simulink model "biquad_filter"  (R2022a)
settings: Solver=FixedStepDiscrete  StartTime=0.0  StopTime=10.0  RelTol=1e-3
PreLoadFcn:
  | addpath('C:\Users\Besic\Documents\MATLAB\hdlimport\biquad_filter');
CloseFcn:
  | addpath('C:\Users\Besic\Documents\MATLAB\hdlimport\biquad_filter');
  | rmpath('C:\Users\Besic\Documents\MATLAB\hdlimport\biquad_filter');
settings Model: DataTypeOverride=Off  Creator=Besic  LastModifiedBy=Besic
settings OptimizationCC: BlockReduction=off  ConditionallyExecuteInputs=off  DefaultParameterBehavior=Inlined  InheritOutputTypeSmallerThanSingle=on
settings DebuggingCC: AlgebraicLoopMsg=error  InheritedTsInSrcMsg=none  SingleTaskRateTransMsg=error
settings HardwareCC: ProdBitPerPointer=32  ProdBitPerSizeT=32  ProdBitPerPtrDiffT=32  ProdLargestAtomicFloat=None  ProdIntDivRoundTo=Undefined  ProdEndianess=Unspecified  ProdWordSize=32  ProdHWDeviceType=ASIC/FPGA->ASIC/FPGA  TargetBitPerPointer=64  TargetBitPerSizeT=64  TargetBitPerPtrDiffT=64  TargetLongLongMode=on  TargetIntDivRoundTo=Zero  TargetEndianess=LittleEndian  TargetWordSize=64  TargetHWDeviceType=Custom Processor->MATLAB Host Computer  ProdEqTarget=off

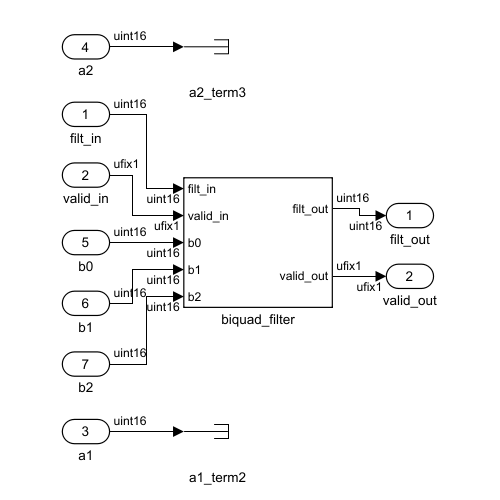
[thumbnail: Simulink's stored preview of the top-level diagram]
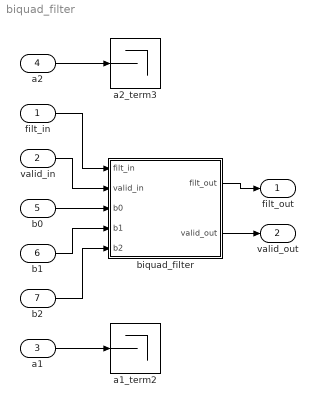
== system biquad_filter ==
  filt_in : Inport  OutDataTypeStr=uint16  SampleTime=-1
  valid_in : Inport  Port=2  OutDataTypeStr=fixdt(0, 1, 0)  SampleTime=-1
  a1 : Inport  Port=3  OutDataTypeStr=uint16  SampleTime=-1
  a2 : Inport  Port=4  OutDataTypeStr=uint16  SampleTime=-1
  b0 : Inport  Port=5  OutDataTypeStr=uint16  SampleTime=-1
  b1 : Inport  Port=6  OutDataTypeStr=uint16  SampleTime=-1
  b2 : Inport  Port=7  OutDataTypeStr=uint16  SampleTime=-1
  a1_term2 : Terminator
  a2_term3 : Terminator
  biquad_filter : Subsystem
  filt_out : Outport  OutDataTypeStr=uint16  SampleTime=-1
  valid_out : Outport  Port=2  OutDataTypeStr=fixdt(0, 1, 0)  SampleTime=-1
  wires:
  a1/1 -> a1_term2/1
  valid_in/1 -> biquad_filter/2(valid_in)
  biquad_filter/2(valid_out) -> valid_out/1
  biquad_filter/1(filt_out) -> filt_out/1
  b2/1 -> biquad_filter/5(b2)
  b1/1 -> biquad_filter/4(b1)
  b0/1 -> biquad_filter/3(b0)
  a2/1 -> a2_term3/1
  filt_in/1 -> biquad_filter/1(filt_in)

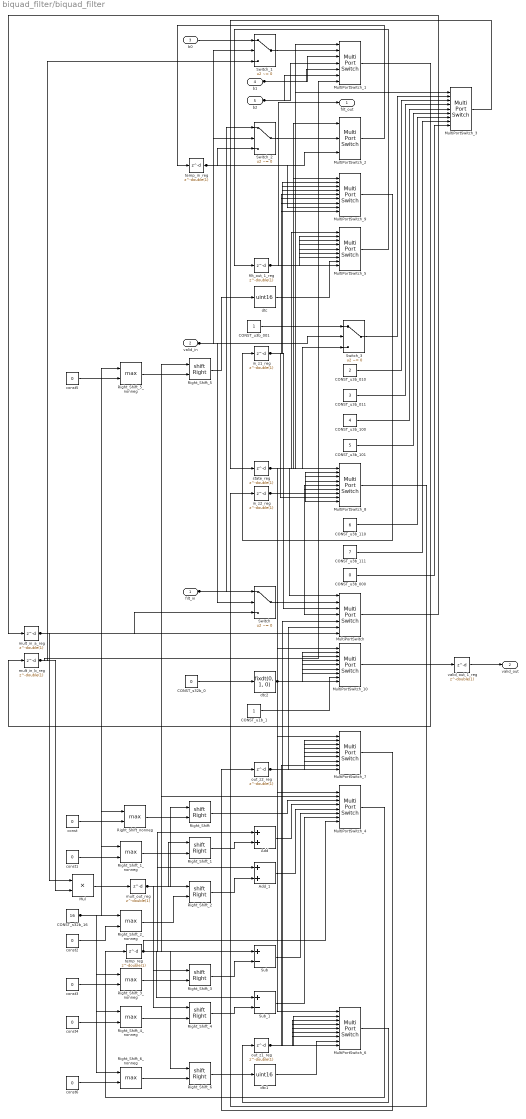
== system biquad_filter/biquad_filter ==
  filt_in : Inport  OutDataTypeStr=uint16  SampleTime=-1
  valid_in : Inport  Port=2  OutDataTypeStr=fixdt(0, 1, 0)  SampleTime=-1
  b0 : Inport  Port=3  OutDataTypeStr=uint16  SampleTime=-1
  b1 : Inport  Port=4  OutDataTypeStr=uint16  SampleTime=-1
  b2 : Inport  Port=5  OutDataTypeStr=uint16  SampleTime=-1
  Add : Sum  AccumDataTypeStr=uint32  OutDataTypeStr=uint32  SampleTime=-1
  Add_1 : Sum  AccumDataTypeStr=uint32  OutDataTypeStr=uint32  SampleTime=-1
  CONST_s32b_0 : Constant  Value=0  OutDataTypeStr=int32  SampleTime=-1
  CONST_s32b_16 : Constant  Value=16  OutDataTypeStr=int32  SampleTime=-1
  CONST_u1b_1 : Constant  OutDataTypeStr=fixdt(0, 1, 0)  SampleTime=-1
  CONST_u3b_000 : Constant  Value=0  OutDataTypeStr=fixdt(0, 3, 0)  SampleTime=-1
  CONST_u3b_001 : Constant  OutDataTypeStr=fixdt(0, 3, 0)  SampleTime=-1
  CONST_u3b_010 : Constant  Value=2  OutDataTypeStr=fixdt(0, 3, 0)  SampleTime=-1
  CONST_u3b_011 : Constant  Value=3  OutDataTypeStr=fixdt(0, 3, 0)  SampleTime=-1
  CONST_u3b_100 : Constant  Value=4  OutDataTypeStr=fixdt(0, 3, 0)  SampleTime=-1
  CONST_u3b_101 : Constant  Value=5  OutDataTypeStr=fixdt(0, 3, 0)  SampleTime=-1
  CONST_u3b_110 : Constant  Value=6  OutDataTypeStr=fixdt(0, 3, 0)  SampleTime=-1
  CONST_u3b_111 : Constant  Value=7  OutDataTypeStr=fixdt(0, 3, 0)  SampleTime=-1
  Mul : Product  Inputs=**  OutDataTypeStr=uint32  SampleTime=-1
  MultiPortSwitch : MultiPortSwitch  DataPortOrder=Zero-based contiguous  Inputs=6  DiagnosticForDefault=None  zeroidx=on  OutDataTypeStr=uint16  SampleTime=-1  SaturateOnIntegerOverflow=off  InputSameDT=off
  MultiPortSwitch_1 : MultiPortSwitch  DataPortOrder=Zero-based contiguous  Inputs=6  DiagnosticForDefault=None  zeroidx=on  OutDataTypeStr=uint16  SampleTime=-1  SaturateOnIntegerOverflow=off  InputSameDT=off
  MultiPortSwitch_10 : MultiPortSwitch  DataPortOrder=Zero-based contiguous  Inputs=8  DiagnosticForDefault=None  zeroidx=on  OutDataTypeStr=fixdt(0, 1, 0)  SampleTime=-1  SaturateOnIntegerOverflow=off  InputSameDT=off
  MultiPortSwitch_2 : MultiPortSwitch  DataPortOrder=Zero-based contiguous  Inputs=2  DiagnosticForDefault=None  zeroidx=on  OutDataTypeStr=uint16  SampleTime=-1  SaturateOnIntegerOverflow=off  InputSameDT=off
  MultiPortSwitch_3 : MultiPortSwitch  DataPortOrder=Zero-based contiguous  Inputs=8  DiagnosticForDefault=None  zeroidx=on  OutDataTypeStr=fixdt(0, 3, 0)  SampleTime=-1  SaturateOnIntegerOverflow=off  InputSameDT=off
  MultiPortSwitch_4 : MultiPortSwitch  DataPortOrder=Zero-based contiguous  Inputs=7  DiagnosticForDefault=None  zeroidx=on  OutDataTypeStr=uint32  SampleTime=-1  SaturateOnIntegerOverflow=off  InputSameDT=off
  MultiPortSwitch_{5..9} (5 alike) : MultiPortSwitch  DataPortOrder=Zero-based contiguous  Inputs=8  DiagnosticForDefault=None  zeroidx=on  OutDataTypeStr=uint16  SampleTime=-1  SaturateOnIntegerOverflow=off  InputSameDT=off
  Right_Shift : ArithShift  BitShiftNumberSource=Input port  BitShiftDirection=Right
      settings: InputPortMap=u0,p1
  Right_Shift_{1..6} (6 alike) : ArithShift  BitShiftNumberSource=Input port  BitShiftDirection=Right
      settings: InputPortMap=u0,p1
  Right_Shift_1_nonneg : MinMax  Function=max  Inputs=2
  Right_Shift_2_nonneg : MinMax  Function=max  Inputs=2
  Right_Shift_3_nonneg : MinMax  Function=max  Inputs=2
  Right_Shift_4_nonneg : MinMax  Function=max  Inputs=2
  Right_Shift_5_nonneg : MinMax  Function=max  Inputs=2
  Right_Shift_6_nonneg : MinMax  Function=max  Inputs=2
  Right_Shift_nonneg : MinMax  Function=max  Inputs=2
  Sub : Sum  Inputs=+-  AccumDataTypeStr=uint32  OutDataTypeStr=uint32  SampleTime=-1
  Sub_1 : Sum  Inputs=+-  AccumDataTypeStr=uint32  OutDataTypeStr=uint32  SampleTime=-1
  Switch : Switch  Criteria=u2 ~= 0  Threshold=double(0)  OutDataTypeStr=uint16  SampleTime=-1  SaturateOnIntegerOverflow=off  InputSameDT=off
  Switch_1 : Switch  Criteria=u2 ~= 0  Threshold=double(0)  OutDataTypeStr=uint16  SampleTime=-1  SaturateOnIntegerOverflow=off  InputSameDT=off
  Switch_2 : Switch  Criteria=u2 ~= 0  Threshold=double(0)  OutDataTypeStr=uint16  SampleTime=-1  SaturateOnIntegerOverflow=off  InputSameDT=off
  Switch_3 : Switch  Criteria=u2 ~= 0  Threshold=double(0)  OutDataTypeStr=fixdt(0, 3, 0)  SampleTime=-1  SaturateOnIntegerOverflow=off  InputSameDT=off
  const{,1..6} (7 alike) : Constant  Value=0  OutDataTypeStr=int32  SampleTime=-1
  dtc : DataTypeConversion  OutDataTypeStr=uint16  SampleTime=-1  SaturateOnIntegerOverflow=off  RndMeth=Floor
  dtc1 : DataTypeConversion  OutDataTypeStr=uint16  SampleTime=-1  SaturateOnIntegerOverflow=off  RndMeth=Floor
  dtc2 : DataTypeConversion  OutDataTypeStr=fixdt(0, 1, 0)  SampleTime=-1  SaturateOnIntegerOverflow=off  RndMeth=Floor
  filt_out_1_reg : Delay  DelayLength=double(1)  InitialCondition=0  SampleTime=-1
  in_z1_reg : Delay  DelayLength=double(1)  InitialCondition=0  SampleTime=-1
  in_z2_reg : Delay  DelayLength=double(1)  InitialCondition=0  SampleTime=-1
  mult_in_a_reg : Delay  DelayLength=double(1)  InitialCondition=0  SampleTime=-1
  mult_in_b_reg : Delay  DelayLength=double(1)  InitialCondition=0  SampleTime=-1
  mult_out_reg : Delay  DelayLength=double(1)  InitialCondition=0  SampleTime=-1
  out_z1_reg : Delay  DelayLength=double(1)  InitialCondition=0  SampleTime=-1
  out_z2_reg : Delay  DelayLength=double(1)  InitialCondition=0  SampleTime=-1
  state_reg : Delay  DelayLength=double(1)  InitialCondition=0  SampleTime=-1
  temp_in_reg : Delay  DelayLength=double(1)  InitialCondition=0  SampleTime=-1
  temp_reg : Delay  DelayLength=double(1)  InitialCondition=0  SampleTime=-1
  valid_out_1_reg : Delay  DelayLength=double(1)  InitialCondition=0  SampleTime=-1
  filt_out : Outport  OutDataTypeStr=uint16  SampleTime=-1
  valid_out : Outport  Port=2  OutDataTypeStr=fixdt(0, 1, 0)  SampleTime=-1
  wires:
  const5/1 -> Right_Shift_5_nonneg/2
  const4/1 -> Right_Shift_4_nonneg/2
  CONST_u3b_100/1 -> MultiPortSwitch_3/5
  const6/1 -> Right_Shift_6_nonneg/2
  in_z1_reg/1 -> MultiPortSwitch_9/9, MultiPortSwitch_9/7, MultiPortSwitch_9/6, MultiPortSwitch_9/5, MultiPortSwitch_9/4, MultiPortSwitch_9/3, MultiPortSwitch_9/2, MultiPortSwitch_8/8, MultiPortSwitch/3
  dtc/1 -> MultiPortSwitch_5/8
  Right_Shift_3_nonneg/1 -> Right_Shift_3/2
  Switch/1 -> MultiPortSwitch/2
  Right_Shift_5_nonneg/1 -> Right_Shift_5/2
  MultiPortSwitch_2/1 -> temp_in_reg/1
  Right_Shift_6_nonneg/1 -> Right_Shift_6/2
  MultiPortSwitch_7/1 -> out_z2_reg/1
  Right_Shift_4_nonneg/1 -> Right_Shift_4/2
  Right_Shift/1 -> MultiPortSwitch_4/3
  const3/1 -> Right_Shift_3_nonneg/2
  MultiPortSwitch_4/1 -> temp_reg/1
  const2/1 -> Right_Shift_2_nonneg/2
  Right_Shift_2_nonneg/1 -> Right_Shift_2/2
  const1/1 -> Right_Shift_1_nonneg/2
  mult_out_reg/1 -> Right_Shift_4/1, Right_Shift_3/1, Right_Shift_2/1, Right_Shift_1/1, Right_Shift/1
  valid_out_1_reg/1 -> valid_out/1
  Switch_1/1 -> MultiPortSwitch_1/2
  CONST_u3b_011/1 -> MultiPortSwitch_3/4
  Right_Shift_1_nonneg/1 -> Right_Shift_1/2
  const/1 -> Right_Shift_nonneg/2
  Right_Shift_nonneg/1 -> Right_Shift/2
  MultiPortSwitch_6/1 -> out_z1_reg/1
  CONST_u1b_1/1 -> MultiPortSwitch_10/8
  Right_Shift_2/1 -> Add_1/2
  Right_Shift_6/1 -> dtc1/1
  dtc1/1 -> MultiPortSwitch_6/8
  Mul/1 -> mult_out_reg/1
  Right_Shift_5/1 -> dtc/1
  Sub_1/1 -> MultiPortSwitch_4/7
  mult_in_b_reg/1 -> Switch_1/3, MultiPortSwitch_1/7, Mul/2
  Right_Shift_4/1 -> Sub_1/2
  CONST_u3b_110/1 -> MultiPortSwitch_3/7
  Sub/1 -> MultiPortSwitch_4/6
  MultiPortSwitch_3/1 -> state_reg/1
  Right_Shift_3/1 -> Sub/2
  Add_1/1 -> MultiPortSwitch_4/5
  CONST_u3b_101/1 -> MultiPortSwitch_3/6
  Add/1 -> MultiPortSwitch_4/4
  MultiPortSwitch/1 -> mult_in_a_reg/1
  Switch_2/1 -> MultiPortSwitch_2/2
  Right_Shift_1/1 -> Add/2
  CONST_u3b_000/1 -> MultiPortSwitch_3/9
  MultiPortSwitch_8/1 -> in_z2_reg/1
  CONST_u3b_111/1 -> MultiPortSwitch_3/8
  CONST_u3b_010/1 -> MultiPortSwitch_3/3
  CONST_u3b_001/1 -> Switch_3/1
  mult_in_a_reg/1 -> Switch/3, MultiPortSwitch/7, Mul/1
  Switch_3/1 -> MultiPortSwitch_3/2
  MultiPortSwitch_9/1 -> in_z1_reg/1
  MultiPortSwitch_1/1 -> mult_in_b_reg/1
  CONST_s32b_0/1 -> dtc2/1
  b0/1 -> Switch_1/1
  MultiPortSwitch_10/1 -> valid_out_1_reg/1
  MultiPortSwitch_5/1 -> filt_out_1_reg/1
  dtc2/1 -> MultiPortSwitch_10/9, MultiPortSwitch_10/7, MultiPortSwitch_10/6, MultiPortSwitch_10/5, MultiPortSwitch_10/4, MultiPortSwitch_10/3, MultiPortSwitch_10/2
  CONST_s32b_16/1 -> Right_Shift_6_nonneg/1, Right_Shift_5_nonneg/1, Right_Shift_4_nonneg/1, Right_Shift_3_nonneg/1, Right_Shift_2_nonneg/1, Right_Shift_1_nonneg/1, Right_Shift_nonneg/1
  out_z2_reg/1 -> MultiPortSwitch_7/9, MultiPortSwitch_7/7, MultiPortSwitch_7/6, MultiPortSwitch_7/5, MultiPortSwitch_7/4, MultiPortSwitch_7/3, MultiPortSwitch_7/2, MultiPortSwitch/6
  out_z1_reg/1 -> MultiPortSwitch_7/8, MultiPortSwitch_6/9, MultiPortSwitch_6/7, MultiPortSwitch_6/6, MultiPortSwitch_6/5, MultiPortSwitch_6/4, MultiPortSwitch_6/3, MultiPortSwitch_6/2, MultiPortSwitch/5
  in_z2_reg/1 -> MultiPortSwitch_8/9, MultiPortSwitch_8/7, MultiPortSwitch_8/6, MultiPortSwitch_8/5, MultiPortSwitch_8/4, MultiPortSwitch_8/3, MultiPortSwitch_8/2, MultiPortSwitch/4
  temp_in_reg/1 -> MultiPortSwitch_9/8, Switch_2/3, MultiPortSwitch_2/3
  temp_reg/1 -> Right_Shift_6/1, Right_Shift_5/1, Sub_1/1, Sub/1, Add_1/1, Add/1, MultiPortSwitch_4/8, MultiPortSwitch_4/2
  state_reg/1 -> MultiPortSwitch_10/1, MultiPortSwitch_9/1, MultiPortSwitch_8/1, MultiPortSwitch_7/1, MultiPortSwitch_6/1, MultiPortSwitch_5/1, MultiPortSwitch_4/1, Switch_3/3, MultiPortSwitch_3/1, MultiPortSwitch_2/1, MultiPortSwitch_1/1, MultiPortSwitch/1
  filt_out_1_reg/1 -> MultiPortSwitch_5/9, MultiPortSwitch_5/7, MultiPortSwitch_5/6, MultiPortSwitch_5/5, MultiPortSwitch_5/4, MultiPortSwitch_5/3, MultiPortSwitch_5/2, filt_out/1
  b2/1 -> MultiPortSwitch_1/6, MultiPortSwitch_1/4
  b1/1 -> MultiPortSwitch_1/5, MultiPortSwitch_1/3
  valid_in/1 -> Switch_3/2, Switch_2/2, Switch_1/2, Switch/2
  filt_in/1 -> Switch_2/1, Switch/1
